simulink model "rate_limiter_and_dynamic_rate_limiter"  (R2021a)
settings: Solver=VariableStepAuto  StartTime=0.0  StopTime=10.0  RelTol=1e-3
libraries: simulink x1
settings Model: Creator=DELL  LastModifiedBy=DELL

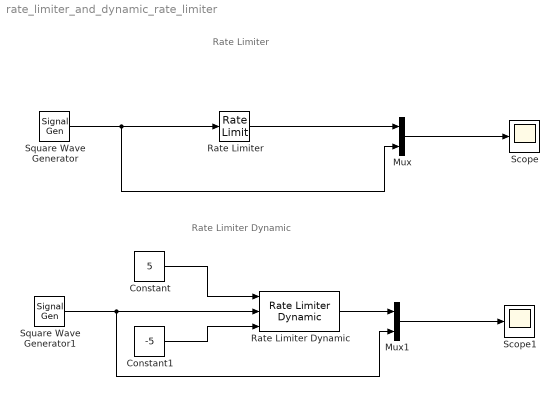
== system rate_limiter_and_dynamic_rate_limiter ==
  note: Rate Limiter
  note: Rate Limiter Dynamic
  Constant : Constant  Value=5
  Constant1 : Constant  Value=-5
  Mux : Mux  Inputs=2
  Mux1 : Mux  Inputs=2
  Rate Limiter : RateLimiter  RisingSlewLimit=5  FallingSlewLimit=-5  SampleTimeMode=inherited
  Rate Limiter Dynamic : simulink/Discontinuities/Rate Limiter Dynamic
  Scope : Scope
  Scope1 : Scope
  Square Wave Generator : SignalGenerator  WaveForm=square  Amplitude=10  Units=rad/sec
  Square Wave Generator1 : SignalGenerator  WaveForm=square  Amplitude=10  Units=rad/sec
  wires:
  Square Wave Generator/1 -> Mux/2, Rate Limiter/1
  Rate Limiter/1 -> Mux/1
  Mux/1 -> Scope/1
  Mux1/1 -> Scope1/1
  Square Wave Generator1/1 -> Rate Limiter Dynamic/2, Mux1/2
  Rate Limiter Dynamic/1 -> Mux1/1
  Constant/1 -> Rate Limiter Dynamic/1
  Constant1/1 -> Rate Limiter Dynamic/3
